simulink model "05.KCU"  (R2019b)
settings: Solver=FixedStepAuto  StartTime=0.0  StopTime=inf  FixedStep=1  MaxStep=1  RelTol=1e-3
libraries: simulink x3
settings Model: Creator=MARAT  LastModifiedBy=Marat
settings SFSimCC: CustomCodeUndefinedFunction=UseInterfaceOnly

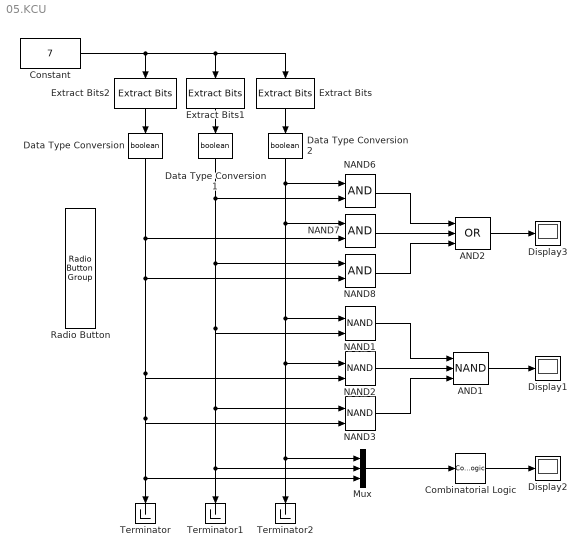
== system 05.KCU ==
  AND1 : Logic  Operator=NAND  Inputs=3  IconShape=distinctive  AllPortsSameDT=off  OutDataTypeStr=boolean
  AND2 : Logic  Operator=OR  Inputs=3  AllPortsSameDT=off  OutDataTypeStr=boolean
  Combinatorial Logic : CombinatorialLogic  TruthTable=[0;0;0;1;0;1;1;1]
  Constant : Constant  Value=7  OutMin=0  OutMax=7  OutDataTypeStr=uint8
  Data Type Conversion : DataTypeConversion  OutDataTypeStr=boolean
  Data Type Conversion1 : DataTypeConversion  OutDataTypeStr=boolean
  Data Type Conversion2 : DataTypeConversion  OutDataTypeStr=boolean
  Display1 : Display
  Display2 : Display
  Display3 : Display
  Extract Bits : simulink/Logic and Bit Operations/Extract Bits  bitsToExtract=Range of bits  numBits=8  bitIdxRange=0  outScalingMode=Treat bit field as an integer
      settings: SourceProductName=Simulink
  Extract Bits1 : simulink/Logic and Bit Operations/Extract Bits  bitsToExtract=Range of bits  numBits=8  bitIdxRange=1  outScalingMode=Treat bit field as an integer
      settings: SourceProductName=Simulink
  Extract Bits2 : simulink/Logic and Bit Operations/Extract Bits  bitsToExtract=Range of bits  numBits=8  bitIdxRange=2  outScalingMode=Treat bit field as an integer
      settings: SourceProductName=Simulink
  Mux : Mux  Inputs=3
  NAND1 : Logic  Operator=NAND  IconShape=distinctive  AllPortsSameDT=off  OutDataTypeStr=boolean
  NAND2 : Logic  Operator=NAND  IconShape=distinctive  AllPortsSameDT=off  OutDataTypeStr=boolean
  NAND3 : Logic  Operator=NAND  IconShape=distinctive  AllPortsSameDT=off  OutDataTypeStr=boolean
  NAND6 : Logic  AllPortsSameDT=off  OutDataTypeStr=boolean
  NAND7 : Logic  AllPortsSameDT=off  OutDataTypeStr=boolean
  NAND8 : Logic  AllPortsSameDT=off  OutDataTypeStr=boolean
  Radio Button : RadioButtonGroup  LabelPosition=Hide  SelectedLabel=7  ButtonGroupName=-
      settings: Values={{'0', '1', '2', '3', '4', '5', '6', '7'}, [0 1 2 3 4 5 6 7]}
  Terminator : Terminator
  Terminator1 : Terminator
  Terminator2 : Terminator
  wires:
  Constant/1 -> Extract Bits/1, Extract Bits1/1, Extract Bits2/1
  Extract Bits/1 -> Data Type Conversion2/1
  Extract Bits1/1 -> Data Type Conversion1/1
  Extract Bits2/1 -> Data Type Conversion/1
  Data Type Conversion/1 -> NAND7/2, NAND8/2, Mux/3, Terminator/1, NAND3/2, NAND2/2
  Data Type Conversion1/1 -> NAND6/2, NAND8/1, Mux/2, Terminator1/1, NAND3/1, NAND1/2
  Data Type Conversion2/1 -> NAND6/1, NAND7/1, Mux/1, Terminator2/1, NAND2/1, NAND1/1
  AND2/1 -> Display3/1
  NAND7/1 -> AND2/2
  NAND8/1 -> AND2/3
  NAND6/1 -> AND2/1
  NAND1/1 -> AND1/1
  NAND3/1 -> AND1/3
  NAND2/1 -> AND1/2
  AND1/1 -> Display1/1
  Mux/1 -> Combinatorial Logic/1
  Combinatorial Logic/1 -> Display2/1
